simulink model "bai2b"  (R2018a)
settings: Solver=ode5  StartTime=0.0  StopTime=20  FixedStep=0.01  RelTol=1e-3
libraries: fuzblock x1
settings Model: Creator=trann  LastModifiedBy=DELL

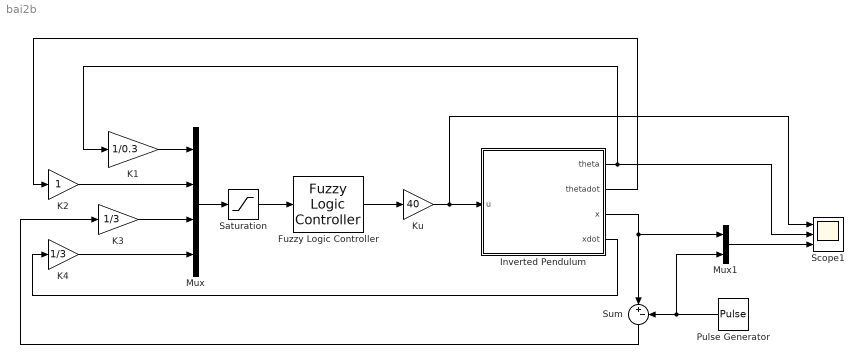
== system bai2b ==
  Fuzzy Logic Controller : fuzblock/Fuzzy Logic  Controller  FIS='fuzz.fis'  OutputSampleNumber=101  DataType=double  FuzzifiedInputs=off  RuleFiringStrengths=off  RuleOutputs=off  AggregatedOutputs=off  SimulateUsing=Interpreted execution  OutOfRangeInputValueMessage=warning  NoRuleFiredMessage=warning  EmptyOutputFuzzySetMessage=warning
  Inverted Pendulum : Subsystem  mask{M1=1.5, m=0.3, g=9.81, l=1}
      mask prompts: M1 "khoi luong xe"; m "khoi luong con lac"; g "gia toc trong truong"; l "chieu dai con lac"
  K1 : Gain  Gain=1/0.3
  K2 : Gain
  K3 : Gain  Gain=1/3
  K4 : Gain  Gain=1/3
  Ku : Gain  Gain=40
  Mux : Mux
  Mux1 : Mux  Inputs=2
  Pulse Generator : DiscretePulseGenerator  PulseType=Time based  Period=20  PulseWidth=50
  Saturation : Saturate  UpperLimit=1  LowerLimit=-1
  Scope1 : Scope  NumInputPorts=3
  Sum : Sum  Inputs=|+-
  wires:
  Fuzzy Logic Controller/1 -> Ku/1
  Mux/1 -> Saturation/1
  Saturation/1 -> Fuzzy Logic Controller/1
  K1/1 -> Mux/1
  K2/1 -> Mux/2
  K3/1 -> Mux/3
  K4/1 -> Mux/4
  Ku/1 -> Scope1/1, Inverted Pendulum/1(u)
  Inverted Pendulum/1(theta) -> K1/1, Scope1/2
  Inverted Pendulum/3(x) -> Mux1/1, Sum/1
  Inverted Pendulum/4(xdot) -> K4/1
  Sum/1 -> K3/1
  Pulse Generator/1 -> Mux1/2, Sum/2
  Inverted Pendulum/2(thetadot) -> K2/1
  Mux1/1 -> Scope1/3

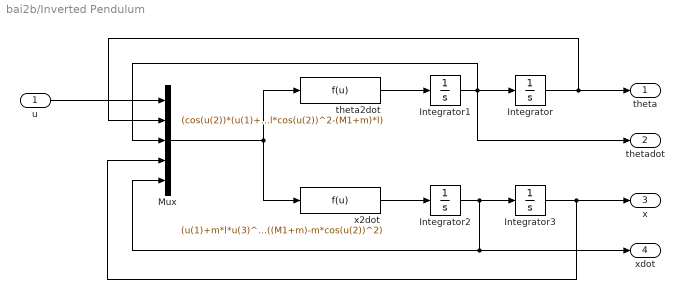
== system bai2b/Inverted Pendulum ==
  u : Inport
  Integrator{,1..3} (4 alike) : Integrator
  Mux : Mux  Inputs=5
  theta2dot : Fcn  Expr=(cos(u(2))*(u(1)+m*g*u(3)^2*sin(u(2)))-(M1+m)*g*sin(u(2)))/(m*l*cos(u(2))^2-(M1+m)*l)
  x2dot : Fcn  Expr=(u(1)+m*l*u(3)^2*sin(u(2))-m*g*sin(u(2))*cos(u(2)))/((M1+m)-m*cos(u(2))^2)
  theta : Outport
  thetadot : Outport  Port=2
  x : Outport  Port=3
  xdot : Outport  Port=4
  wires:
  Mux/1 -> theta2dot/1, x2dot/1
  u/1 -> Mux/1
  Integrator3/1 -> Mux/4, x/1
  x2dot/1 -> Integrator2/1
  theta2dot/1 -> Integrator1/1
  Integrator1/1 -> thetadot/1, Mux/3, Integrator/1
  Integrator2/1 -> Mux/5, xdot/1, Integrator3/1
  Integrator/1 -> Mux/2, theta/1
